simulink model "BallBeam"  (R2014b)
settings: Solver=ode45  StartTime=0.0  StopTime=200  RelTol=1e-3
undefined symbols (not defined in the file or in its folder): Kp, Td
settings Model: Creator=jeff  LastModifiedBy=jeff

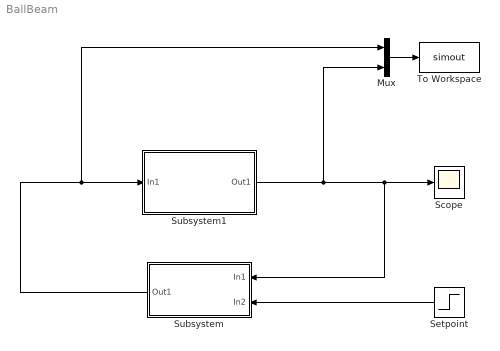
== system BallBeam ==
  Mux : Mux  Inputs=2
  Scope : Scope
  Setpoint : Step  Time=20  SampleTime=0
  Subsystem : Subsystem
  Subsystem1 : Subsystem
  To Workspace : ToWorkspace  VariableName=simout  SaveFormat=Timeseries  SampleTime=-1
  wires:
  Setpoint/1 -> Subsystem/2(In2)
  Subsystem1/1(Out1) -> Mux/2, Subsystem/1(In1), Scope/1
  Subsystem/1(Out1) -> Mux/1, Subsystem1/1(In1)
  Mux/1 -> To Workspace/1

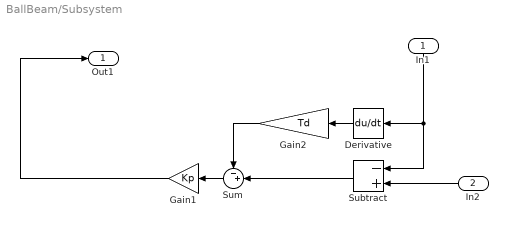
== system BallBeam/Subsystem ==
  In1 : Inport
  In2 : Inport  Port=2
  Derivative : Derivative
  Gain1 : Gain  Gain=Kp
  Gain2 : Gain  Gain=Td
  Subtract : Sum  Inputs=-+
  Sum : Sum  Inputs=-+|
  Out1 : Outport
  wires:
  Derivative/1 -> Gain2/1
  Subtract/1 -> Sum/2
  In2/1 -> Subtract/2
  In1/1 -> Derivative/1, Subtract/1
  Gain1/1 -> Out1/1
  Gain2/1 -> Sum/1
  Sum/1 -> Gain1/1

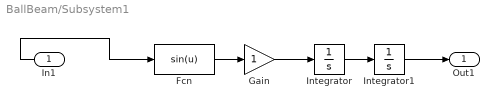
== system BallBeam/Subsystem1 ==
  In1 : Inport
  Fcn : Fcn  Expr=sin(u)
  Gain : Gain
  Integrator : Integrator
  Integrator1 : Integrator
  Out1 : Outport
  wires:
  Fcn/1 -> Gain/1
  Integrator/1 -> Integrator1/1
  Integrator1/1 -> Out1/1
  In1/1 -> Fcn/1
  Gain/1 -> Integrator/1
